simulink model "TPS_Logic_Stateflow"  (R2020a)
settings: Solver=FixedStepDiscrete  StartTime=0.0  StopTime=10.0  FixedStep=.1  RelTol=1e-3
settings Model: Creator=Administrator  LastModifiedBy=Administrator
settings OptimizationCC: DefaultParameterBehavior=Inlined  EnhancedBackFolding=on  PassReuseOutputArgsAs=Individual arguments  ZeroExternalMemoryAtStartup=off  ZeroInternalMemoryAtStartup=off  OptimizeBlockOrder=speed  DifferentSizesBufferReuse=on  OptimizationCustomize=off  EfficientTunableParamExpr=on
settings DebuggingCC: ParameterTunabilityLossMsg=error
settings HardwareCC: ProdBitPerPointer=32  ProdBitPerSizeT=32  ProdBitPerPtrDiffT=32  ProdLargestAtomicInteger=Long  ProdLargestAtomicFloat=Double  ProdWordSize=32  ProdHWDeviceType=ARM Compatible->ARM Cortex
settings SFSimCC: MATLABDynamicMemAlloc=off
settings RTWCC: SystemTargetFile=ert.tlc  GenCodeOnly=on  TemplateMakefile=ert_default_tmf
settings CodeAppCC: ForceParamTrailComments=on  IgnoreCustomStorageClasses=off  OperatorAnnotations=on  SimulinkDataObjDesc=on  SFDataObjDesc=on  InsertBlockDesc=on
settings ERTTargetCC: TargetLangStandard=C99 (ISO)  GenerateSampleERTMain=on  InlinedParameterPlacement=NonHierarchical  ERTCustomFileTemplate=example_file_process.tlc

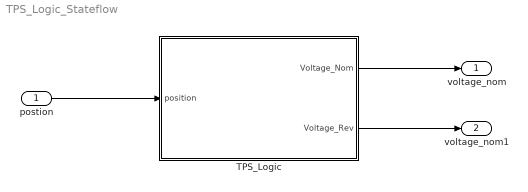
== system TPS_Logic_Stateflow ==
  postion : Inport
  TPS_Logic : Stateflow chart  TreatAsAtomicUnit=on
  voltage_nom : Outport
  voltage_nom1 : Outport  Port=2
  wires:
  postion/1 -> TPS_Logic/1(position)
  TPS_Logic/1(Voltage_Nom) -> voltage_nom/1
  TPS_Logic/2(Voltage_Rev) -> voltage_nom1/1

== stateflow chart TPS_Logic_Stateflow/TPS_Logic ==
  state System_Handle
    state TPS_RevSen_Voltage [parallel]
      en:
      Voltage_Rev=(position*(-2*pi))+4.5;
      settings: executionOrder=1
    state TPS_Sen_Voltage [parallel]
      en:
      Voltage_Nom=(position*(2*pi))+.5;
      settings: executionOrder=2
    TPS_RevSen_Voltage -> TPS_RevSen_Voltage
    TPS_Sen_Voltage -> TPS_Sen_Voltage
  data: position input; Voltage_Nom output; Voltage_Rev output
